simulink model "f14autopilot"  (Simulink 6.0)
settings: Solver=ode45  SolverMode=SingleTasking  StartTime=0.0  StopTime=10.0  RelTol=1e-3  AbsTol=1e-6
values from neighbouring files (symbols this model uses):
  Ka = 0.6770    (= 0.677)    [f14dat.m]    (also in f14dat_digital.m; f14def.m)
  Kf = -1.7460    (= -1.746)    [f14dat.m]    (also in f14dat_digital.m; f14def.m)
  Ki = -3.8640    (= -3.864)    [f14dat.m]    (also in f14dat_digital.m; f14def.m)
  Kq = 0.8156    [f14dat.m]    (also in f14dat_digital.m; f14def.m)
  Tal = 0.3959    [f14dat.m]    (also in f14dat_digital.m; f14def.m)
  Ts = 0.1000    (= 0.1)    [f14dat.m]    (also in f14dat_digital.m; f14def.m)
  W1 = 2.9710    (= 2.971)    [f14dat.m]    (also in f14dat_digital.m; f14def.m)
  W2 = 4.1440    (= 4.144)    [f14dat.m]    (also in f14dat_digital.m; f14def.m)
libraries: slctrlobsolete x4
settings Model: Creator=The MathWorks Inc.  LastModifiedBy=batserve  ExtModeTrigMode=oneshot  ExtModeArmWhenConnect=off  ExtModeAutoUpdateStatusClock=off
settings DataIOCC: LimitDataPoints=off  SignalLoggingName=logsOut
settings OptimizationCC: BooleanDataType=off
settings DebuggingCC: CheckExecutionContextPreStartOutputMsg=on  CheckExecutionContextRuntimeOutputMsg=on  SolverPrmCheckMsg=none  IntegerOverflowMsg=none
settings HardwareCC: TargetUnknown=on
settings RTWCC: TemplateMakefile=grt_vc.tmf

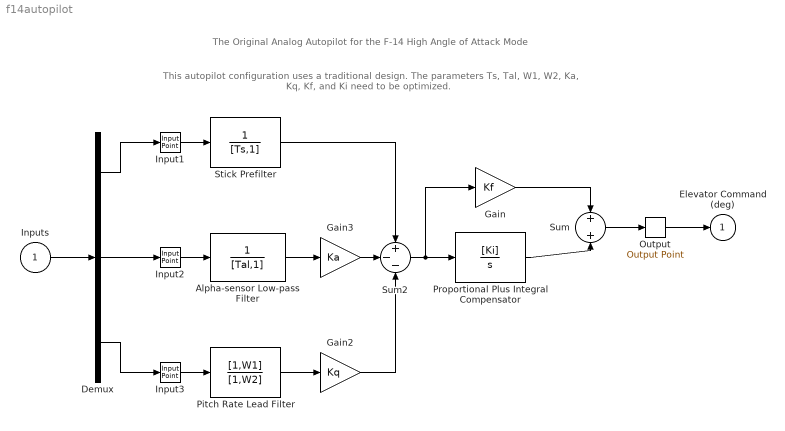
== system f14autopilot ==
  note: The Original Analog Autopilot for the F-14 High Angle of Attack Mode
  note: This autopilot configuration uses a traditional design.
      | The parameters Ts, Tal, W1, W2, Ka, Kq, Kf, and Ki need to be optimized.
  Inputs : Inport  Port=1  PortDimensions=3  LatchInput=off
  Alpha-sensor Low-pass Filter : TransferFcn  Denominator=[Tal,1]
  Demux : Demux  Outputs=3
  Gain : Gain  Gain=Kf  SaturateOnIntegerOverflow=on
  Gain2 : Gain  Gain=Kq  SaturateOnIntegerOverflow=on
  Gain3 : Gain  Gain=Ka  SaturateOnIntegerOverflow=on
  Input1 : slctrlobsolete/Input Point
  Input2 : slctrlobsolete/Input Point
  Input3 : slctrlobsolete/Input Point
  Output : slctrlobsolete/Output Point
  Pitch Rate Lead Filter : TransferFcn  Numerator=[1,W1]  Denominator=[1,W2]
  Proportional Plus Integral Compensator : TransferFcn  Numerator=[Ki]  Denominator=[1,0]
  Stick Prefilter : TransferFcn  Denominator=[Ts,1]
  Sum : Sum  Inputs=2  SaturateOnIntegerOverflow=on  InputSameDT=on
  Sum2 : Sum  Inputs=+--  SaturateOnIntegerOverflow=on  InputSameDT=on
  Elevator Command (deg) : Outport  InitialOutput=0
  wires:
  Input1/1 -> Stick Prefilter/1
  Stick Prefilter/1 -> Sum2/1
  Pitch Rate Lead Filter/1 -> Gain2/1
  Alpha-sensor Low-pass Filter/1 -> Gain3/1
  Gain3/1 -> Sum2/2
  Gain2/1 -> Sum2/3
  Inputs/1 -> Demux/1
  Sum2/1 -> Proportional Plus Integral Compensator/1, Gain/1
  Gain/1 -> Sum/1
  Proportional Plus Integral Compensator/1 -> Sum/2
  Demux/1 -> Input1/1
  Demux/2 -> Input2/1
  Input2/1 -> Alpha-sensor Low-pass Filter/1
  Demux/3 -> Input3/1
  Input3/1 -> Pitch Rate Lead Filter/1
  Sum/1 -> Output/1
  Output/1 -> Elevator Command (deg)/1
